simulink model "floatingball"  (R2016a)
settings: Solver=VariableStepAuto  StartTime=0.0  StopTime=10  RelTol=1e-3
libraries: simulink x2
settings Model: Creator=13  LastModifiedBy=rafael
settings SolverCC: MaxConsecutiveMinStep=10

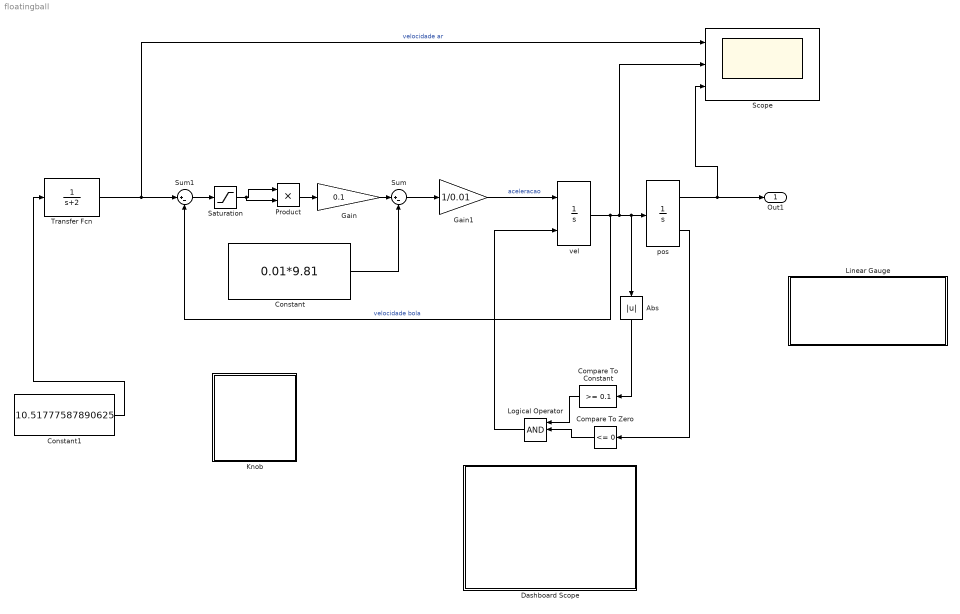
== system floatingball ==
  Abs : Abs
  Compare To Constant : simulink/Logic and Bit Operations/Compare To Constant  relop=>=  const=0.1  OutDataTypeStr=boolean
  Compare To Zero : simulink/Logic and Bit Operations/Compare To Zero  relop=<=  OutDataTypeStr=boolean
  Constant : Constant  Value=0.01*9.81
  Constant1 : Constant  Value=10.51777587890625
  Dashboard Scope : Subsystem  DialogController=hmiCreateDDGDialog  IsWebBlock=on  mask(MWDashboardBlock){webBlockId=ff3d8f0a-9521-4646-be61-4fdb8ec1a734, webBlockType=sdiscope, ShowInitialText=on, HMISrcModelName=floatingball}
      mask prompts: webBlockId "WebBlock Id"; webBlockType "WebBlock Type"; HMISrcModelName "Source Model"
      mask Help: helpview([docroot '/mapfiles/simulink.map'], 'hmi_scope')
      mask Display:
      | if strcmp(get_param(bdroot(gcb),'BlockDiagramType'), 'library')
      |     image([(matlabroot) '/toolbox/simulink/hmi/icons/DashboardScope.png']);
      | end
  Gain : Gain  Gain=0.1
  Gain1 : Gain  Gain=1/0.01
  Knob : Subsystem  DialogController=hmiCreateDDGDialog  IsWebBlock=on  mask(MWDashboardBlock){webBlockId=4063064d-cc54-4609-805f-29b09b23701f, webBlockType=continuousknob, ShowInLibBrowser=on, ShowInitialText=on, HMISrcModelName=floatingball}
      mask prompts: webBlockId "WebBlock Id"; webBlockType "WebBlock Type"; HMISrcModelName "Source Model"
      mask Help: helpview([docroot '/mapfiles/simulink.map'], 'hmi_knob')
      mask Display:
      | if strcmp(get_param(bdroot(gcb),'BlockDiagramType'), 'library')
      |     image([(matlabroot) '/toolbox/simulink/hmi/icons/ContinuousKnob.png']);
      | end
  Linear Gauge : Subsystem  DialogController=hmiCreateDDGDialog  IsWebBlock=on  mask(MWDashboardBlock){webBlockId=b1e92d02-fcc5-46ba-9cb1-703f2b1f59c9, webBlockType=lineargauge, ShowInLibBrowser=on, ShowInitialText=on, HMISrcModelName=floatingball}
      mask prompts: webBlockId "WebBlock Id"; webBlockType "WebBlock Type"; HMISrcModelName "Source Model"
      mask Help: helpview([docroot '/mapfiles/simulink.map'], 'hmi_linear_gauge')
      mask Display:
      | if strcmp(get_param(bdroot(gcb),'BlockDiagramType'), 'library')
      |     image([(matlabroot) '/toolbox/simulink/hmi/icons/LinearGauge.png']);
      | end
  Logical Operator : Logic  Inputs=3  AllPortsSameDT=off  OutDataTypeStr=boolean
  Product : Product
  Saturation : Saturate  UpperLimit=Inf  LowerLimit=0
  Scope : Scope  NumInputPorts=3
  Sum : Sum  Inputs=|+-
  Sum1 : Sum  Inputs=|+-
  Transfer Fcn : TransferFcn  Denominator=[1 2]
  "pos " : Integrator  InitialCondition=1e-3  LimitOutput=on  UpperSaturationLimit=40e-2  LowerSaturationLimit=0  ShowSaturationPort=on
  vel : Integrator  ExternalReset=rising  LimitOutput=on  UpperSaturationLimit=30  LowerSaturationLimit=-30
  Out1 : Outport  PortDimensions=1
  wires:
  Transfer Fcn/1 -> Scope/1, Sum1/1  "velocidade ar"
  vel/1 -> Sum1/2, Scope/2, Abs/1, "pos "/1  "velocidade bola"
  Constant/1 -> Sum/2
  Gain/1 -> Sum/1
  Sum/1 -> Gain1/1
  Gain1/1 -> vel/1  "aceleracao"
  Constant1/1 -> Transfer Fcn/1
  "pos "/1 -> Scope/3, Out1/1
  "pos "/2 -> Compare To Zero/1
  Product/1 -> Gain/1
  Sum1/1 -> Saturation/1
  Abs/1 -> Compare To Constant/1
  Logical Operator/1 -> vel/2
  Compare To Constant/1 -> Logical Operator/1
  Compare To Zero/1 -> Logical Operator/2
  Saturation/1 -> Product/2, Product/1

== system floatingball/Dashboard Scope ==

== system floatingball/Knob ==

== system floatingball/Linear Gauge ==
